simulink model "UbicacionDePolos"  (R2017a)
settings: Solver=VariableStepAuto  StartTime=0.0  StopTime=10.0  RelTol=1e-3
settings Model: Creator=Jesus  LastModifiedBy=Jesus

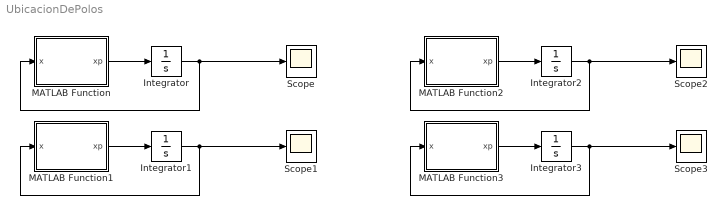
== system UbicacionDePolos ==
  Integrator{,1..3} (4 alike) : Integrator  InitialCondition=[0 0]
  MATLAB Function : MATLAB Function  TreatAsAtomicUnit=on
  MATLAB Function1 : MATLAB Function  TreatAsAtomicUnit=on
  MATLAB Function2 : MATLAB Function  TreatAsAtomicUnit=on
  MATLAB Function3 : MATLAB Function  TreatAsAtomicUnit=on
  Scope{,1..3} (4 alike) : Scope
  wires:
  MATLAB Function/1(xp) -> Integrator/1
  Integrator/1 -> Scope/1, MATLAB Function/1(x)
  Integrator1/1 -> MATLAB Function1/1(x), Scope1/1
  MATLAB Function1/1(xp) -> Integrator1/1
  MATLAB Function3/1(xp) -> Integrator3/1
  Integrator3/1 -> Scope3/1, MATLAB Function3/1(x)
  Integrator2/1 -> MATLAB Function2/1(x), Scope2/1
  MATLAB Function2/1(xp) -> Integrator2/1

== matlab function UbicacionDePolos/MATLAB Function1 ==
  data: x input; xp output
function xp = fcn(x)
r=1;
K=[4,5.6667];
u=r-K*x;
A = [1 3;3 1];
B = [1 0]';
xp = A*x+B*u;

== matlab function UbicacionDePolos/MATLAB Function ==
  data: x input; xp output
function xp = fcn(x)
u=1;
A = [1 3;3 1];
B = [1 0]';
xp = A*x+B*u;

== matlab function UbicacionDePolos/MATLAB Function2 ==
  data: x input; xp output
function xp = fcn(x)
u=1;
A = [1 3;3 1];
B = [1 0]';
xp = A*x+B*u;

== matlab function UbicacionDePolos/MATLAB Function3 ==
  data: x input; xp output
function xp = fcn(x)
r=1;
K=[3.5,4];
u=r-K*x;
A = [1 3;3 1];
B = [1 0]';
xp = A*x+B*u;
